simulink model "QCwithActDyn"  (R2019b)
settings: Solver=FixedStepAuto  StartTime=0.0  StopTime=15  FixedStep=0.001  RelTol=1e-3
model workspace (MAT data in the model file):
  time_step = 0.01
libraries: simulink x1
settings Model: Creator=Abdulaziz Y. Alkayas  LastModifiedBy=aaa_b
settings SolverCC: SolverResetMethod=Robust
settings DebuggingCC: ArithmeticOperatorsInVariantConditions=warning
settings HardwareCC: TargetBitPerPointer=64  TargetBitPerSizeT=64  TargetBitPerPtrDiffT=64  TargetLongLongMode=on  TargetIntDivRoundTo=Zero  TargetEndianess=LittleEndian  TargetWordSize=64  TargetHWDeviceType=MATLAB Host  ProdEqTarget=off
settings SFSimCC: CustomCodeUndefinedFunction=UseInterfaceOnly
settings RTWCC: Description=Generic Real-Time Target

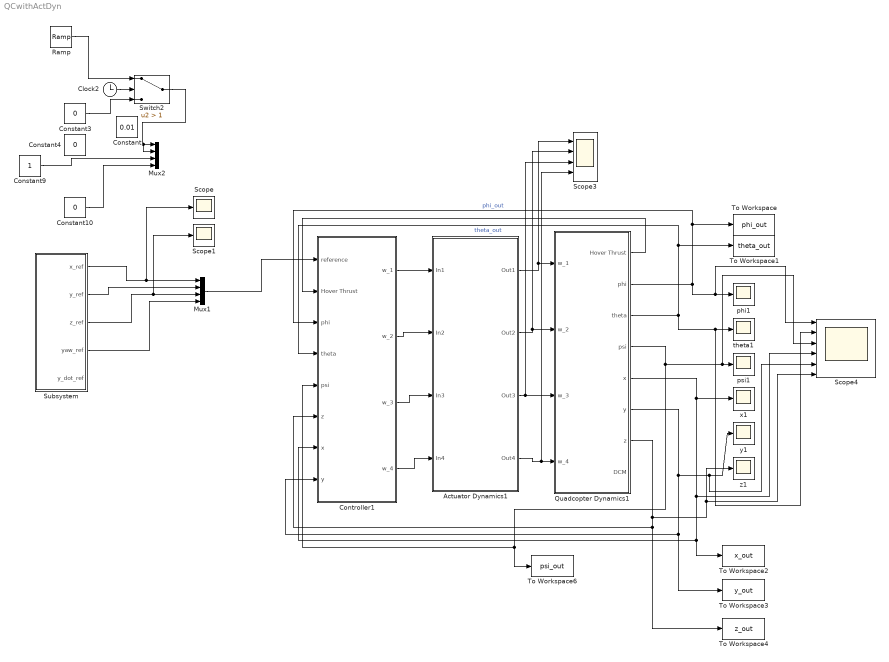
== system QCwithActDyn ==
  Actuator Dynamics1 : Subsystem
  Clock2 : Clock
  Constant : Constant  Value=0.01
  Constant10 : Constant  Value=0
  Constant3 : Constant  Value=0
  Constant4 : Constant  Value=0
  Constant9 : Constant
  Controller1 : Subsystem
  Mux1 : Mux
  Mux2 : Mux
  Quadcopter Dynamics1 : Subsystem
  Ramp : simulink/Sources/Ramp  slope=1  start=2  InitialOutput=0
  Scope : Scope
  Scope1 : Scope
  Scope3 : Scope  NumInputPorts=4
  Scope4 : Scope  NumInputPorts=6
  Subsystem : Subsystem
  Switch2 : Switch  Criteria=u2 > Threshold  Threshold=1
  To Workspace : ToWorkspace  VariableName=phi_out  SaveFormat=Timeseries  SampleTime=-1
  To Workspace1 : ToWorkspace  VariableName=theta_out  SaveFormat=Timeseries  SampleTime=-1
  To Workspace2 : ToWorkspace  VariableName=x_out  SaveFormat=Timeseries  SampleTime=-1
  To Workspace3 : ToWorkspace  VariableName=y_out  SaveFormat=Timeseries  SampleTime=-1
  To Workspace4 : ToWorkspace  VariableName=z_out  SaveFormat=Timeseries  SampleTime=-1
  To Workspace6 : ToWorkspace  VariableName=psi_out  SaveFormat=Timeseries  SampleTime=-1
  phi1 : Scope
  psi1 : Scope
  theta1 : Scope
  x1 : Scope
  y1 : Scope
  z1 : Scope
  wires:
  Controller1/4(w_4) -> Actuator Dynamics1/4(In4)
  Controller1/3(w_3) -> Actuator Dynamics1/3(In3)
  Controller1/2(w_2) -> Actuator Dynamics1/2(In2)
  Controller1/1(w_1) -> Actuator Dynamics1/1(In1)
  Quadcopter Dynamics1/3(theta) -> theta1/1, Scope4/2, To Workspace1/1, Controller1/4(theta)  "theta_out"
  Quadcopter Dynamics1/2(phi) -> Controller1/3(phi), To Workspace/1, phi1/1, Scope4/1  "phi_out"
  Quadcopter Dynamics1/4(psi) -> To Workspace6/1, Controller1/5(psi), psi1/1, Scope4/3
  Quadcopter Dynamics1/7(z) -> To Workspace4/1, Controller1/6(z), z1/1, Scope4/6
  Quadcopter Dynamics1/1(Hover Thrust) -> Controller1/2(Hover Thrust)
  Quadcopter Dynamics1/5(x) -> Scope4/4, To Workspace2/1, Controller1/7(x), x1/1
  Quadcopter Dynamics1/6(y) -> To Workspace3/1, Controller1/8(y), y1/1, Scope4/5
  Ramp/1 -> Switch2/1
  Constant9/1 -> Mux2/3
  Constant10/1 -> Mux2/4
  Clock2/1 -> Switch2/2
  Constant3/1 -> Switch2/3
  Subsystem/4("yaw_ref ") -> Mux1/4
  Subsystem/1("x_ref ") -> Mux1/1, Scope/1
  Switch2/1 -> Mux2/2, Mux2/1
  Mux1/1 -> Controller1/1(reference)
  Subsystem/3("z_ref ") -> Scope1/1, Mux1/3
  Actuator Dynamics1/1(Out1) -> Scope3/1, Quadcopter Dynamics1/1(w_1)
  Actuator Dynamics1/2(Out2) -> Quadcopter Dynamics1/2(w_2), Scope3/2
  Actuator Dynamics1/3(Out3) -> Quadcopter Dynamics1/3(w_3), Scope3/3
  Actuator Dynamics1/4(Out4) -> Quadcopter Dynamics1/4(w_4), Scope3/4
  Subsystem/2("y_ref ") -> Mux1/2

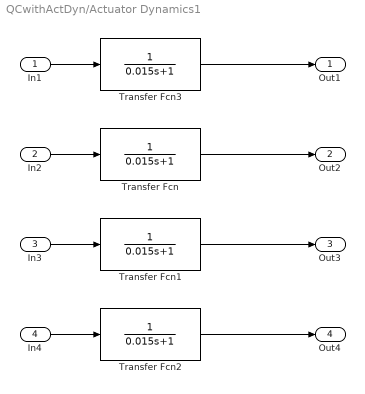
== system QCwithActDyn/Actuator Dynamics1 ==
  In1 : Inport
  In2 : Inport  Port=2
  In3 : Inport  Port=3
  In4 : Inport  Port=4
  Transfer Fcn{,1..3} (4 alike) : TransferFcn  Denominator=[0.015 1]
  Out1 : Outport
  Out2 : Outport  Port=2
  Out3 : Outport  Port=3
  Out4 : Outport  Port=4
  wires:
  In4/1 -> Transfer Fcn2/1
  Transfer Fcn2/1 -> Out4/1
  Transfer Fcn1/1 -> Out3/1
  In2/1 -> Transfer Fcn/1
  Transfer Fcn/1 -> Out2/1
  Transfer Fcn3/1 -> Out1/1
  In3/1 -> Transfer Fcn1/1
  In1/1 -> Transfer Fcn3/1

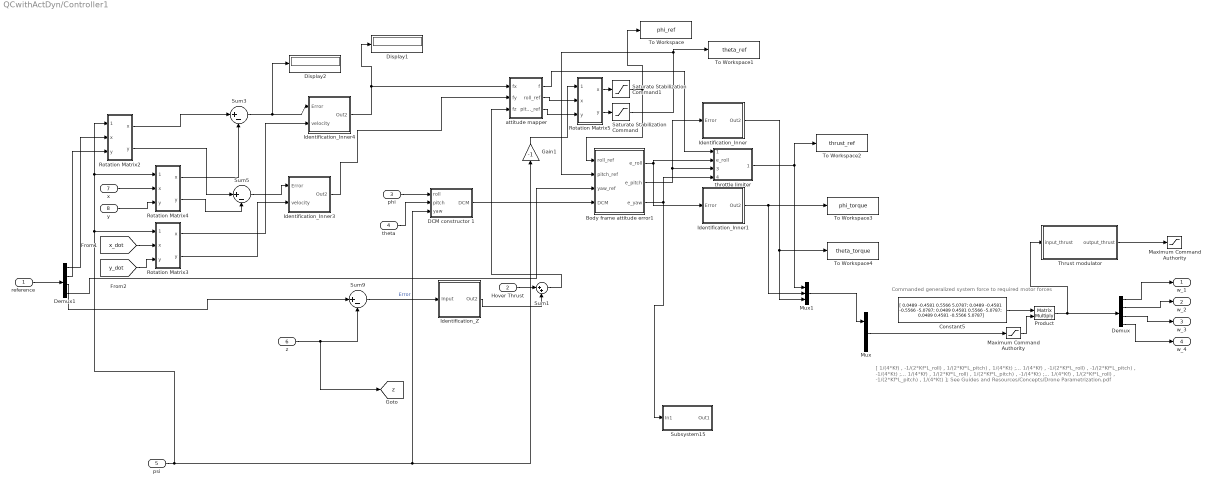
== system QCwithActDyn/Controller1 ==
  note: [ 1/(4*Kf) , -1/(2*Kf*L_roll) , 1/(2*Kf*L_pitch) , 1/(4*Kt) ;...
      | 1/(4*Kf) , -1/(2*Kf*L_roll) , -1/(2*Kf*L_pitch) , -1/(4*Kt) ;...
      | 1/(4*Kf) , 1/(2*Kf*L_roll) , 1/(2*Kf*L_pitch) , -1/(4*Kt) ;...
      | 1/(4*Kf) , 1/(2*Kf*L_roll) , -1/(2*Kf*L_pitch) , 1/(4*Kt) ];
      |
      | See Guides and Resources/Concepts/Drone Parametrization.pdf
  note: Commanded generalized system force to required motor forces
  reference : Inport
  Hover Thrust : Inport  Port=2
  phi : Inport  Port=3
  theta : Inport  Port=4
  psi : Inport  Port=5
  z : Inport  Port=6
  x : Inport  Port=7
  y : Inport  Port=8
  Body frame attitude error1 : MATLAB Function  TreatAsAtomicUnit=on
  Constant5 : Constant  Value=|
      | [ 0.0489   -0.4581    0.5566    5.0787;
      |   0.0489   -0.4581   -0.5566   -5.0787;
      |   0.0489    0.4581    0.5566   -5.0787;
      |   0.0489    0.4581   -0.5566    5.0787]
  DCM constructor 1 : MATLAB Function  TreatAsAtomicUnit=on
  Demux : Demux
  Demux1 : Demux
  Display1 : Display
  Display2 : Display
  Gain1 : Gain  Gain=-1
  Identification_Inner : Subsystem
  Identification_Inner1 : Subsystem
  Identification_Inner3 : Subsystem
  Identification_Inner4 : Subsystem
  Identification_Z : Subsystem
  Maximum Command Authority : Saturate  UpperLimit=[Inf Inf Inf Inf]  LowerLimit=[-inf -Inf -Inf -Inf]
  "Maximum Command Authority " : Saturate  UpperLimit=[1 1 1 1]  LowerLimit=[0 0 0 0]
  Mux : Mux  Inputs=[3, 1]
  Mux1 : Mux  Inputs=3
  Product : Product  Multiplication=Matrix(*)
  Rotation Matrix2 : Subsystem
  Rotation Matrix3 : Subsystem
  Rotation Matrix4 : Subsystem
  Rotation Matrix5 : Subsystem
  Saturate Stabilization Command : Saturate  UpperLimit=pi/2  LowerLimit=-pi/2
  Saturate Stabilization Command1 : Saturate  UpperLimit=pi/2  LowerLimit=-pi/2
  Subsystem15 : Subsystem
  Sum1 : Sum  Inputs=|++
  Sum3 : Sum  Inputs=|+-
  Sum5 : Sum  Inputs=|+-
  Sum9 : Sum  Inputs=|+-
  Thrust modulator : MATLAB Function  TreatAsAtomicUnit=on
  To Workspace : ToWorkspace  VariableName=phi_ref  SaveFormat=Timeseries  SampleTime=-1
  To Workspace1 : ToWorkspace  VariableName=theta_ref  SaveFormat=Timeseries  SampleTime=-1
  To Workspace2 : ToWorkspace  VariableName=thrust_ref  SaveFormat=Timeseries  SampleTime=-1
  To Workspace3 : ToWorkspace  VariableName=phi_torque  SaveFormat=Timeseries  SampleTime=-1
  To Workspace4 : ToWorkspace  VariableName=theta_torque  SaveFormat=Timeseries  SampleTime=-1
  "attitude mapper " : MATLAB Function  TreatAsAtomicUnit=on
  throttle limiter : MATLAB Function  TreatAsAtomicUnit=on
  w_1 : Outport
  w_2 : Outport  Port=2
  w_3 : Outport  Port=3
  w_4 : Outport  Port=4
  tag scope: z=global
  wires:
  z/1 -> Sum9/2, [z]
  Maximum Command Authority/1 -> Product/2
  Mux/1 -> Maximum Command Authority/1
  Constant5/1 -> Product/1
  Demux/2 -> w_2/1
  Demux/3 -> w_3/1
  Demux/4 -> w_4/1
  Sum3/1 -> Display2/1, Identification_Inner4/1(Error)
  Sum5/1 -> Identification_Inner3/1(Error)
  Hover Thrust/1 -> Sum1/1
  Demux/1 -> w_1/1
  Sum9/1 -> Identification_Z/1(Input)  "Error"
  Identification_Z/1(Out2) -> Sum1/2
  reference/1 -> Demux1/1
  Demux1/3 -> Sum9/1
  Identification_Inner4/1(Out2) -> Display1/1, "attitude mapper "/1(fx)
  Identification_Inner3/1(Out2) -> "attitude mapper "/2(fy)
  Sum1/1 -> "attitude mapper "/3(fz)
  Demux1/4 -> Body frame attitude error1/3(yaw_ref)
  Body frame attitude error1/3(e_yaw) -> throttle limiter/4(e_yaw), Subsystem15/1(In1)
  Body frame attitude error1/2(e_pitch) -> Identification_Inner/1(Error), throttle limiter/3(e_pitch)
  Body frame attitude error1/1(e_roll) -> Identification_Inner1/1(Error), throttle limiter/2(e_roll)
  Demux1/1 -> Rotation Matrix2/2("x ")
  Demux1/2 -> Rotation Matrix2/3(y)
  Rotation Matrix2/1(x) -> Sum3/1
  Rotation Matrix2/2("y ") -> Sum5/1
  [x_dot] -> Rotation Matrix3/2("x ")
  [y_dot] -> Rotation Matrix3/3(y)
  Rotation Matrix3/1(x) -> Identification_Inner4/2("velocity ")
  Rotation Matrix3/2("y ") -> Identification_Inner3/2("velocity ")
  x/1 -> Rotation Matrix4/2("x ")
  y/1 -> Rotation Matrix4/3(y)
  Rotation Matrix4/1(x) -> Sum3/2
  Rotation Matrix4/2("y ") -> Sum5/2
  DCM constructor 1/1(DCM) -> Body frame attitude error1/4(DCM)
  "attitude mapper "/2(roll_ref) -> Rotation Matrix5/2("x ")
  "attitude mapper "/3(pitch_ref) -> Rotation Matrix5/3(y)
  Rotation Matrix5/1(x) -> Saturate Stabilization Command1/1
  Identification_Inner1/1(Out2) -> Mux1/2, To Workspace3/1
  Identification_Inner/1(Out2) -> Mux1/3, To Workspace4/1
  Mux1/1 -> Mux/1
  psi/1 -> Rotation Matrix4/1("yaw "), Rotation Matrix2/1("yaw "), Rotation Matrix3/1("yaw "), Gain1/1, DCM constructor 1/3(yaw)
  Gain1/1 -> Rotation Matrix5/1("yaw ")
  Rotation Matrix5/2("y ") -> Saturate Stabilization Command/1
  Saturate Stabilization Command/1 -> To Workspace1/1, Body frame attitude error1/2(pitch_ref)
  Saturate Stabilization Command1/1 -> To Workspace/1, Body frame attitude error1/1(roll_ref)
  phi/1 -> DCM constructor 1/1(roll)
  theta/1 -> DCM constructor 1/2(pitch)
  "attitude mapper "/1(f) -> throttle limiter/1(throttle_in)
  throttle limiter/1(throttle_out) -> Mux1/1, To Workspace2/1
  Product/1 -> Thrust modulator/1(input_thrust), Demux/1
  Thrust modulator/1(output_thrust) -> "Maximum Command Authority "/1

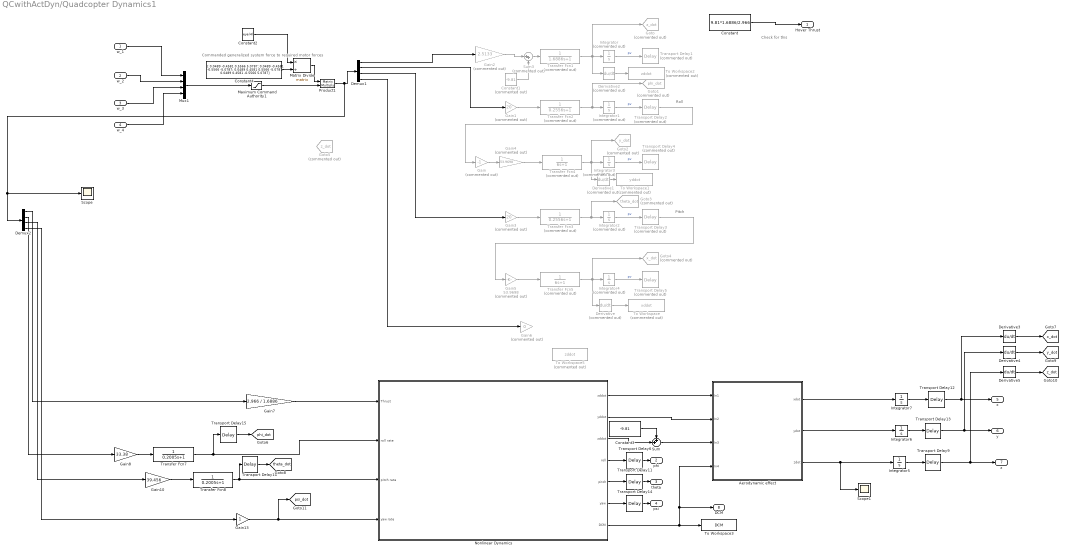
== system QCwithActDyn/Quadcopter Dynamics1 ==
  note: Check for this
  note: Pitch
  note: Roll
  note: Commanded generalized system force to required motor forces
  w_1 : Inport
  w_2 : Inport  Port=2
  w_3 : Inport  Port=3
  w_4 : Inport  Port=4
  "Aerodynamic effect " : Subsystem
  Constant : Constant  Value=9.81*1.6886/2.966
  Constant1 : Constant  Commented=on  Value=-9.81
  Constant2 : Constant  Value=eye(4)
  Constant3 : Constant  Value=-9.81
  Constant4 : Constant  Value=|
      | [ 0.0489   -0.4581    0.5566    5.0787;
      |   0.0489   -0.4581   -0.5566   -5.0787;
      |   0.0489    0.4581    0.5566   -5.0787;
      |   0.0489    0.4581   -0.5566    5.0787]
  Demux1 : Demux
  Demux2 : Demux
  Derivative : Derivative  Commented=on
  Derivative1 : Derivative  Commented=on
  Derivative2 : Derivative  Commented=on
  Derivative3 : Derivative
  Derivative4 : Derivative
  Derivative5 : Derivative
  Gain : Gain  Commented=on  Gain=-1
  Gain1 : Gain  Commented=on  Gain=20
  Gain10 : Gain  Gain=39.456
  Gain13 : Gain
  Gain2 : Gain  Commented=on  Gain=2.5133
  Gain3 : Gain  Commented=on  Gain=20
  Gain4 : Gain  Commented=on  Gain=53.9698
  Gain5 : Gain  Commented=on  Gain=53.9698
  Gain6 : Gain  Commented=on  Gain=0
  Gain7 : Gain  Gain=2.966 / 1.6886
  Gain8 : Gain  Gain=33.38
  Goto : Goto  Commented=on  GotoTag=z_dot  TagVisibility=global
  Goto1 : Goto  Commented=on  GotoTag=phi_dot  TagVisibility=global
  Goto2 : Goto  Commented=on  GotoTag=y_dot  TagVisibility=global
  Goto3 : Goto  Commented=on  GotoTag=theta_dot  TagVisibility=global
  Goto4 : Goto  Commented=on  GotoTag=x_dot  TagVisibility=global
  Goto5 : Goto  Commented=on  GotoTag=z_dot  TagVisibility=global
  Integrator{,1..4} (5 alike) : Integrator  Commented=on
  Integrator5 : Integrator
  Integrator6 : Integrator
  Integrator7 : Integrator  InitialCondition=-3
  Matrix Divide : Product  Inputs=*/  Multiplication=Matrix(*)
  Maximum Command Authority1 : Saturate  UpperLimit=[Inf Inf Inf Inf]  LowerLimit=[-Inf -Inf -Inf -Inf]
  Mux1 : Mux
  Nonlinear Dynamics : Subsystem
  Product1 : Product  Multiplication=Matrix(*)
  Scope : Scope
  Scope1 : Scope
  Sum : Sum  Inputs=++|
  Sum3 : Sum  Commented=on  Inputs=|++
  To Workspace : ToWorkspace  Commented=on  VariableName=xddot  SaveFormat=Timeseries  SampleTime=-1
  To Workspace1 : ToWorkspace  Commented=on  VariableName=yddot  SaveFormat=Timeseries  SampleTime=-1
  To Workspace2 : ToWorkspace  Commented=on  VariableName=zddot  SaveFormat=Timeseries  SampleTime=-1
  To Workspace3 : ToWorkspace  VariableName=DCM  SaveFormat=Timeseries  SampleTime=-1
  To Workspace5 : ToWorkspace  Commented=on  VariableName=zddot  SaveFormat=Timeseries  SampleTime=-1
  Transfer Fcn1 : TransferFcn  Commented=on  Denominator=[1.6886 1]
  Transfer Fcn2 : TransferFcn  Commented=on  Denominator=[0.2556 1]
  Transfer Fcn3 : TransferFcn  Commented=on  Denominator=[0.2556 1]
  Transfer Fcn4 : TransferFcn  Commented=on  Denominator=[6 1]
  Transfer Fcn5 : TransferFcn  Commented=on  Denominator=[6 1]
  Transfer Fcn7 : TransferFcn  Denominator=[0.2005 1]
  Transfer Fcn8 : TransferFcn  Denominator=[0.2005 1]
  Transport Delay1 : TransportDelay  Commented=on  DelayTime=0.0237
  Transport Delay{6,11,15..16} (4 alike) : TransportDelay  DelayTime=0.025
  Transport Delay12 : TransportDelay  DelayTime=0.0223  InitialOutput=-3
  Transport Delay13 : TransportDelay  DelayTime=0.0223
  Transport Delay14 : TransportDelay  DelayTime=0.01
  Transport Delay2 : TransportDelay  Commented=on  DelayTime=0.0180
  Transport Delay3 : TransportDelay  Commented=on  DelayTime=0.0180
  Transport Delay4 : TransportDelay  Commented=on  DelayTime=0.0223
  Transport Delay5 : TransportDelay  Commented=on  DelayTime=0.0223
  Transport Delay9 : TransportDelay  DelayTime=0.027
  Hover Thrust : Outport
  phi : Outport  Port=2
  theta : Outport  Port=3
  psi : Outport  Port=4
  x : Outport  Port=5
  y : Outport  Port=6
  z : Outport  Port=7
  DCM : Outport  Port=8
  tag scope: phi_dot=global, psi_dot=global, theta_dot=global, x_dot=global, y_dot=global, z_dot=global
  wires:
  Transfer Fcn1/1 -> Derivative2/1, Goto/1, Integrator/1
  Integrator/1 -> Transport Delay1/1  "pv"
  Integrator1/1 -> Transport Delay2/1  "pv"
  Transfer Fcn2/1 -> Goto1/1, Integrator1/1
  Gain1/1 -> Transfer Fcn2/1
  Transport Delay2/1 -> Gain/1
  Gain3/1 -> Transfer Fcn3/1
  Transfer Fcn3/1 -> Goto3/1, Integrator2/1
  Integrator2/1 -> Transport Delay3/1  "pv"
  Transport Delay3/1 -> Gain5/1
  Demux1/2 -> Gain1/1
  Demux1/3 -> Gain3/1
  Integrator3/1 -> Transport Delay4/1  "pv"
  Gain5/1 -> Transfer Fcn5/1
  Transfer Fcn5/1 -> Derivative/1, Goto4/1, Integrator4/1
  Sum3/1 -> Transfer Fcn1/1
  Integrator4/1 -> Transport Delay5/1  "pv"
  Demux1/4 -> Gain6/1
  w_2/1 -> Mux1/2
  w_3/1 -> Mux1/3
  w_4/1 -> Mux1/4
  Maximum Command Authority1/1 -> Product1/2
  Constant2/1 -> Matrix Divide/1
  Mux1/1 -> Maximum Command Authority1/1
  Constant4/1 -> Matrix Divide/2
  w_1/1 -> Mux1/1
  Demux1/1 -> Gain2/1
  Constant1/1 -> Sum3/2
  Gain2/1 -> Sum3/1
  Gain/1 -> Gain4/1
  Transfer Fcn4/1 -> Derivative1/1, Goto2/1, Integrator3/1
  Gain4/1 -> Transfer Fcn4/1
  Derivative/1 -> To Workspace/1
  Derivative1/1 -> To Workspace1/1
  Derivative2/1 -> To Workspace2/1
  Nonlinear Dynamics/1(xddot) -> "Aerodynamic effect "/1(In1)
  Nonlinear Dynamics/2(yddot) -> "Aerodynamic effect "/2(In2)
  Nonlinear Dynamics/7(DCM) -> To Workspace3/1, "Aerodynamic effect "/4(In4), DCM/1
  Integrator7/1 -> Transport Delay12/1
  Demux2/4 -> Gain13/1
  Demux2/3 -> Gain10/1
  Demux2/2 -> Gain8/1
  Transfer Fcn8/1 -> Transport Delay16/1, Nonlinear Dynamics/3(pitch rate)
  Gain10/1 -> Transfer Fcn8/1
  Gain8/1 -> Transfer Fcn7/1
  Nonlinear Dynamics/4(roll) -> Transport Delay6/1
  Nonlinear Dynamics/5("pitch ") -> Transport Delay11/1
  "Aerodynamic effect "/1("xdot ") -> Integrator7/1
  "Aerodynamic effect "/2(ydot) -> Integrator6/1
  Nonlinear Dynamics/3(zddot) -> Sum/2
  Sum/1 -> "Aerodynamic effect "/3(In3)
  Transport Delay11/1 -> theta/1
  Transport Delay6/1 -> phi/1
  Integrator5/1 -> Transport Delay9/1
  Transport Delay12/1 -> Derivative3/1, x/1
  Integrator6/1 -> Transport Delay13/1
  Transfer Fcn7/1 -> Transport Delay15/1, Nonlinear Dynamics/2("roll rate ")
  "Aerodynamic effect "/3(zdot) -> Scope1/1, Integrator5/1
  Constant3/1 -> Sum/1
  Constant/1 -> Hover Thrust/1
  Demux2/1 -> Gain7/1
  Transport Delay14/1 -> psi/1
  Nonlinear Dynamics/6(yaw) -> Transport Delay14/1
  Transport Delay15/1 -> [phi_dot]
  Transport Delay16/1 -> [theta_dot]
  Gain13/1 -> [psi_dot], Nonlinear Dynamics/4("yaw rate ")
  Gain7/1 -> Nonlinear Dynamics/1(Thrust)
  Derivative5/1 -> [z_dot]
  Derivative4/1 -> [y_dot]
  Transport Delay9/1 -> Derivative5/1, z/1
  Derivative3/1 -> [x_dot]
  Transport Delay13/1 -> Derivative4/1, y/1
  Product1/1 -> Scope/1, Demux2/1, Demux1/1
  Matrix Divide/1 -> Product1/1

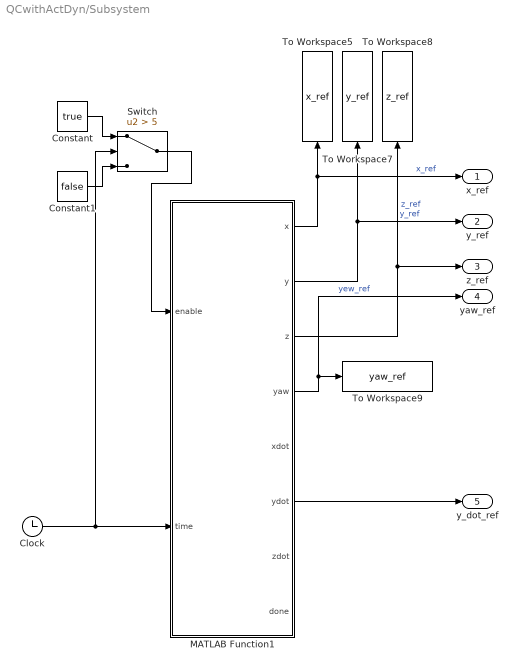
== system QCwithActDyn/Subsystem ==
  Clock : Clock
  Constant : Constant  Value=true
  Constant1 : Constant  Value=false
  MATLAB Function1 : MATLAB Function  TreatAsAtomicUnit=on
  Switch : Switch  Criteria=u2 > Threshold  Threshold=5
  To Workspace5 : ToWorkspace  VariableName=x_ref  SaveFormat=Timeseries  SampleTime=-1
  To Workspace7 : ToWorkspace  VariableName=y_ref  SaveFormat=Timeseries  SampleTime=-1
  To Workspace8 : ToWorkspace  VariableName=z_ref  SaveFormat=Timeseries  SampleTime=-1
  To Workspace9 : ToWorkspace  VariableName=yaw_ref  SaveFormat=Timeseries  SampleTime=-1
  "x_ref " : Outport
  "y_ref " : Outport  Port=2
  "z_ref " : Outport  Port=3
  "yaw_ref " : Outport  Port=4
  "y_dot_ref " : Outport  Port=5
  wires:
  Switch/1 -> MATLAB Function1/1(enable)
  Clock/1 -> Switch/2, MATLAB Function1/2(time)
  MATLAB Function1/3(z) -> To Workspace8/1, "z_ref "/1  "z_ref"
  MATLAB Function1/1(x) -> "x_ref "/1, To Workspace5/1  "x_ref"
  MATLAB Function1/2(y) -> "y_ref "/1, To Workspace7/1  "y_ref"
  MATLAB Function1/4(yaw) -> "yaw_ref "/1, To Workspace9/1  "yew_ref"
  Constant/1 -> Switch/1
  Constant1/1 -> Switch/3
  MATLAB Function1/6(ydot) -> "y_dot_ref "/1

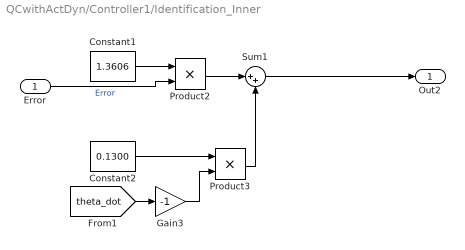
== system QCwithActDyn/Controller1/Identification_Inner ==
  Error : Inport
  Constant1 : Constant  Value=1.3606
  Constant2 : Constant  Value=0.1300
  Gain3 : Gain  Gain=-1
  Product2 : Product
  Product3 : Product
  Sum1 : Sum  Inputs=|++
  Out2 : Outport
  wires:
  Error/1 -> Product2/2  "Error"
  [theta_dot] -> Gain3/1
  Product2/1 -> Sum1/1
  Constant2/1 -> Product3/1
  Gain3/1 -> Product3/2
  Constant1/1 -> Product2/1
  Sum1/1 -> Out2/1
  Product3/1 -> Sum1/2

== system QCwithActDyn/Controller1/Identification_Inner1 ==
  Error : Inport
  Constant3 : Constant  Value=1.6910
  Constant4 : Constant  Value=0.1615
  Gain3 : Gain  Gain=-1
  Product2 : Product
  Product3 : Product
  Sum1 : Sum  Inputs=|++
  Out2 : Outport
  wires:
  Sum1/1 -> Out2/1
  Product3/1 -> Sum1/2
  Constant4/1 -> Product3/1
  Constant3/1 -> Product2/1
  [phi_dot] -> Gain3/1
  Gain3/1 -> Product3/2
  Product2/1 -> Sum1/1
  Error/1 -> Product2/2  "Error"

== system QCwithActDyn/Controller1/Identification_Inner3 ==
  Error : Inport
  "velocity " : Inport  Port=2
  Constant3 : Constant  Value=20.5475
  Constant4 : Constant  Value=6.8752
  Product2 : Product
  Product3 : Product
  Sum : Sum  Inputs=|-+
  Sum1 : Sum  Inputs=|++
  Out2 : Outport
  wires:
  Product2/1 -> Sum1/1
  Constant4/1 -> Product3/1
  Sum/1 -> Product3/2
  Constant3/1 -> Product2/1
  Sum1/1 -> Out2/1
  Product3/1 -> Sum1/2
  "velocity "/1 -> Sum/1  "Error"
  Error/1 -> Product2/2  "Error"

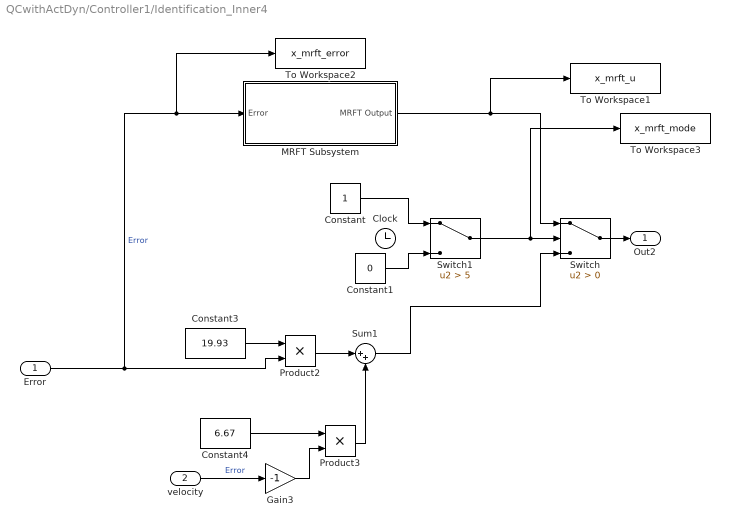
== system QCwithActDyn/Controller1/Identification_Inner4 ==
  Error : Inport
  "velocity " : Inport  Port=2
  Clock : Clock
  Constant : Constant
  Constant1 : Constant  Value=0
  Constant3 : Constant  Value=19.93
  Constant4 : Constant  Value=6.67
  Gain3 : Gain  Gain=-1
  MRFT Subsystem : Subsystem
  Product2 : Product
  Product3 : Product
  Sum1 : Sum  Inputs=|++
  Switch : Switch  Criteria=u2 > Threshold
  Switch1 : Switch  Criteria=u2 > Threshold  Threshold=5
  To Workspace1 : ToWorkspace  VariableName=x_mrft_u  SaveFormat=Timeseries  SampleTime=0.001
  To Workspace2 : ToWorkspace  VariableName=x_mrft_error  SaveFormat=Timeseries  SampleTime=0.001
  To Workspace3 : ToWorkspace  VariableName=x_mrft_mode  SaveFormat=Timeseries  SampleTime=0.001
  Out2 : Outport
  wires:
  Error/1 -> Product2/2, To Workspace2/1, MRFT Subsystem/1(Error)  "Error"
  Product2/1 -> Sum1/1
  Constant4/1 -> Product3/1
  Gain3/1 -> Product3/2
  Constant3/1 -> Product2/1
  Product3/1 -> Sum1/2
  Constant1/1 -> Switch1/3
  Constant/1 -> Switch1/1
  MRFT Subsystem/1(MRFT Output) -> To Workspace1/1, Switch/1
  Switch1/1 -> To Workspace3/1, Switch/2
  Sum1/1 -> Switch/3
  Switch/1 -> Out2/1
  "velocity "/1 -> Gain3/1  "Error"

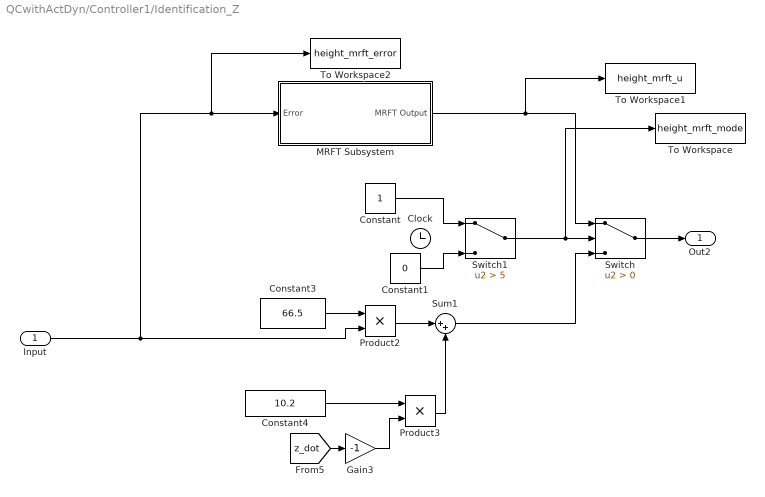
== system QCwithActDyn/Controller1/Identification_Z ==
  Input : Inport
  Clock : Clock
  Constant : Constant
  Constant1 : Constant  Value=0
  Constant3 : Constant  Value=66.5
  Constant4 : Constant  Value=10.2
  Gain3 : Gain  Gain=-1
  MRFT Subsystem : Subsystem
  Product2 : Product
  Product3 : Product
  Sum1 : Sum  Inputs=|++
  Switch : Switch  Criteria=u2 > Threshold
  Switch1 : Switch  Criteria=u2 > Threshold  Threshold=5
  To Workspace : ToWorkspace  VariableName=height_mrft_mode  SaveFormat=Timeseries  SampleTime=0.001
  To Workspace1 : ToWorkspace  VariableName=height_mrft_u  SaveFormat=Timeseries  SampleTime=0.001
  To Workspace2 : ToWorkspace  VariableName=height_mrft_error  SaveFormat=Timeseries  SampleTime=0.001
  Out2 : Outport
  wires:
  Constant4/1 -> Product3/1
  Gain3/1 -> Product3/2
  Product3/1 -> Sum1/2
  [z_dot] -> Gain3/1
  Product2/1 -> Sum1/1
  Constant3/1 -> Product2/1
  Input/1 -> To Workspace2/1, MRFT Subsystem/1(Error), Product2/2
  Switch/1 -> Out2/1
  Switch1/1 -> To Workspace/1, Switch/2
  Sum1/1 -> Switch/3
  MRFT Subsystem/1(MRFT Output) -> To Workspace1/1, Switch/1
  Constant1/1 -> Switch1/3
  Constant/1 -> Switch1/1

== system QCwithActDyn/Controller1/Rotation Matrix2 ==
  "yaw " : Inport
  "x " : Inport  Port=2
  y : Inport  Port=3
  reference correction : MATLAB Function  TreatAsAtomicUnit=on
  x : Outport
  "y " : Outport  Port=2
  wires:
  "yaw "/1 -> reference correction/1(yaw)
  "x "/1 -> reference correction/2(x)
  y/1 -> reference correction/3(y)
  reference correction/1(x_out) -> x/1
  reference correction/2(y_out) -> "y "/1

== system QCwithActDyn/Controller1/Rotation Matrix3 ==
  "yaw " : Inport
  "x " : Inport  Port=2
  y : Inport  Port=3
  reference correction : MATLAB Function  TreatAsAtomicUnit=on
  x : Outport
  "y " : Outport  Port=2
  wires:
  reference correction/2(y_out) -> "y "/1
  reference correction/1(x_out) -> x/1
  y/1 -> reference correction/3(y)
  "x "/1 -> reference correction/2(x)
  "yaw "/1 -> reference correction/1(yaw)

== system QCwithActDyn/Controller1/Rotation Matrix4 ==
  "yaw " : Inport
  "x " : Inport  Port=2
  y : Inport  Port=3
  reference correction : MATLAB Function  TreatAsAtomicUnit=on
  x : Outport
  "y " : Outport  Port=2
  wires:
  "yaw "/1 -> reference correction/1(yaw)
  "x "/1 -> reference correction/2(x)
  y/1 -> reference correction/3(y)
  reference correction/1(x_out) -> x/1
  reference correction/2(y_out) -> "y "/1

== system QCwithActDyn/Controller1/Rotation Matrix5 ==
  "yaw " : Inport
  "x " : Inport  Port=2
  y : Inport  Port=3
  reference correction : MATLAB Function  TreatAsAtomicUnit=on
  x : Outport
  "y " : Outport  Port=2
  wires:
  "yaw "/1 -> reference correction/1(yaw)
  "x "/1 -> reference correction/2(x)
  y/1 -> reference correction/3(y)
  reference correction/1(x_out) -> x/1
  reference correction/2(y_out) -> "y "/1

== system QCwithActDyn/Controller1/Subsystem15 ==
  In1 : Inport
  Gain2 : Gain  Gain=0.12
  Gain3 : Gain  Gain=0.6
  Sum6 : Sum  Inputs=|-+
  Out1 : Outport
  wires:
  Gain3/1 -> Sum6/2
  Gain2/1 -> Sum6/1
  Sum6/1 -> Out1/1
  In1/1 -> Gain3/1
  [psi_dot] -> Gain2/1

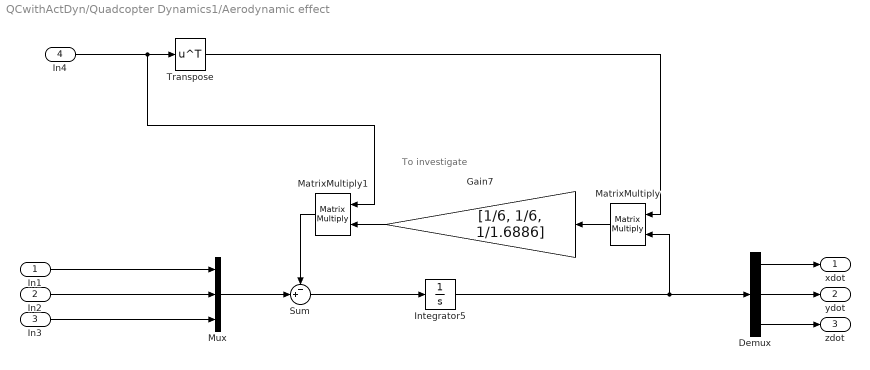
== system QCwithActDyn/Quadcopter Dynamics1/Aerodynamic effect  ==
  note: To investigate
  In1 : Inport
  In2 : Inport  Port=2
  In3 : Inport  Port=3
  In4 : Inport  Port=4
  Demux : Demux  Outputs=3
  Gain7 : Gain  Gain=[1/6, 1/6, 1/1.6886]
  Integrator5 : Integrator
  MatrixMultiply : Product  Multiplication=Matrix(*)
  MatrixMultiply1 : Product  Multiplication=Matrix(*)
  Mux : Mux  Inputs=3
  Sum : Sum  Inputs=-+|
  Transpose : Math  Operator=transpose  SignedPower=off  SaturateOnIntegerOverflow=on
  "xdot " : Outport
  ydot : Outport  Port=2
  zdot : Outport  Port=3
  wires:
  Mux/1 -> Sum/2
  In3/1 -> Mux/3
  MatrixMultiply/1 -> Gain7/1
  In2/1 -> Mux/2
  In1/1 -> Mux/1
  Demux/1 -> "xdot "/1
  Demux/2 -> ydot/1
  Demux/3 -> zdot/1
  Integrator5/1 -> MatrixMultiply/2, Demux/1
  Gain7/1 -> MatrixMultiply1/2
  Transpose/1 -> MatrixMultiply/1
  In4/1 -> MatrixMultiply1/1, Transpose/1
  Sum/1 -> Integrator5/1
  MatrixMultiply1/1 -> Sum/1

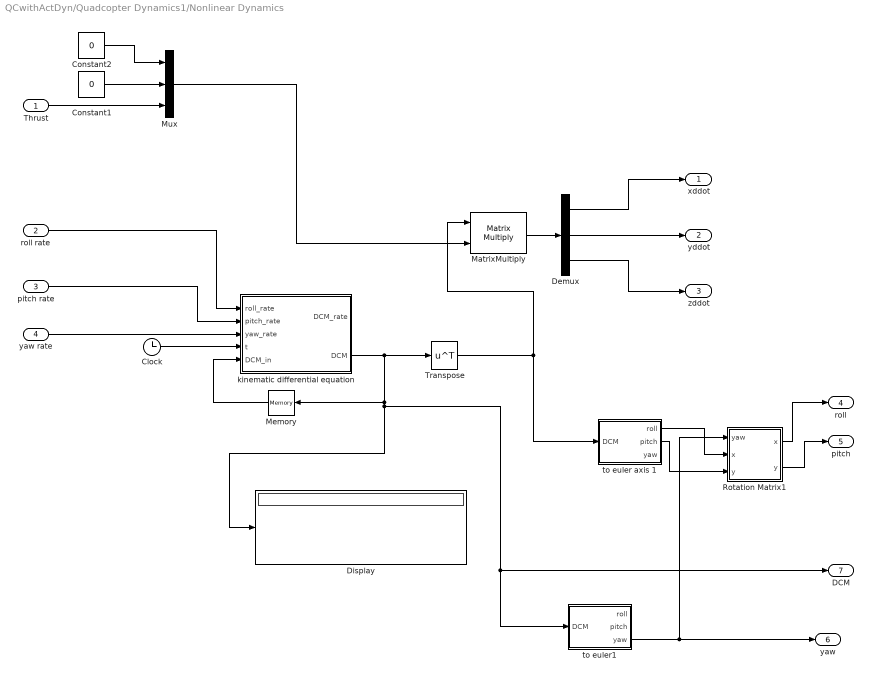
== system QCwithActDyn/Quadcopter Dynamics1/Nonlinear Dynamics ==
  Thrust : Inport
  "roll rate " : Inport  Port=2
  pitch rate : Inport  Port=3
  "yaw rate " : Inport  Port=4
  Clock : Clock
  Constant1 : Constant  Value=0
  Constant2 : Constant  Value=0
  Demux : Demux  Outputs=3
  Display : Display
  MatrixMultiply : Product  Multiplication=Matrix(*)
  Memory : Memory  InitialCondition=eye(3)
  Mux : Mux  Inputs=3
  Rotation Matrix1 : Subsystem
  Transpose : Math  Operator=transpose  SignedPower=off  SaturateOnIntegerOverflow=on
  kinematic differential equation : MATLAB Function  TreatAsAtomicUnit=on
  to euler axis 1 : MATLAB Function  TreatAsAtomicUnit=on
  to euler1 : MATLAB Function  TreatAsAtomicUnit=on
  xddot : Outport
  yddot : Outport  Port=2
  zddot : Outport  Port=3
  roll : Outport  Port=4
  "pitch " : Outport  Port=5
  yaw : Outport  Port=6
  DCM : Outport  Port=7
  wires:
  "yaw rate "/1 -> kinematic differential equation/3(yaw_rate)
  Thrust/1 -> Mux/3
  Constant2/1 -> Mux/1
  Constant1/1 -> Mux/2
  Mux/1 -> MatrixMultiply/2
  MatrixMultiply/1 -> Demux/1
  Demux/1 -> xddot/1
  Demux/2 -> yddot/1
  Demux/3 -> zddot/1
  "roll rate "/1 -> kinematic differential equation/1(roll_rate)
  pitch rate/1 -> kinematic differential equation/2(pitch_rate)
  Transpose/1 -> MatrixMultiply/1, to euler axis 1/1(DCM)
  to euler1/3(yaw) -> Rotation Matrix1/1("yaw "), yaw/1
  kinematic differential equation/2(DCM) -> Memory/1, to euler1/1(DCM), DCM/1, Display/1, Transpose/1
  Clock/1 -> kinematic differential equation/4(t)
  Memory/1 -> kinematic differential equation/5(DCM_in)
  to euler axis 1/1(roll) -> Rotation Matrix1/2("x ")
  to euler axis 1/2(pitch) -> Rotation Matrix1/3(y)
  Rotation Matrix1/2("y ") -> "pitch "/1
  Rotation Matrix1/1(x) -> roll/1

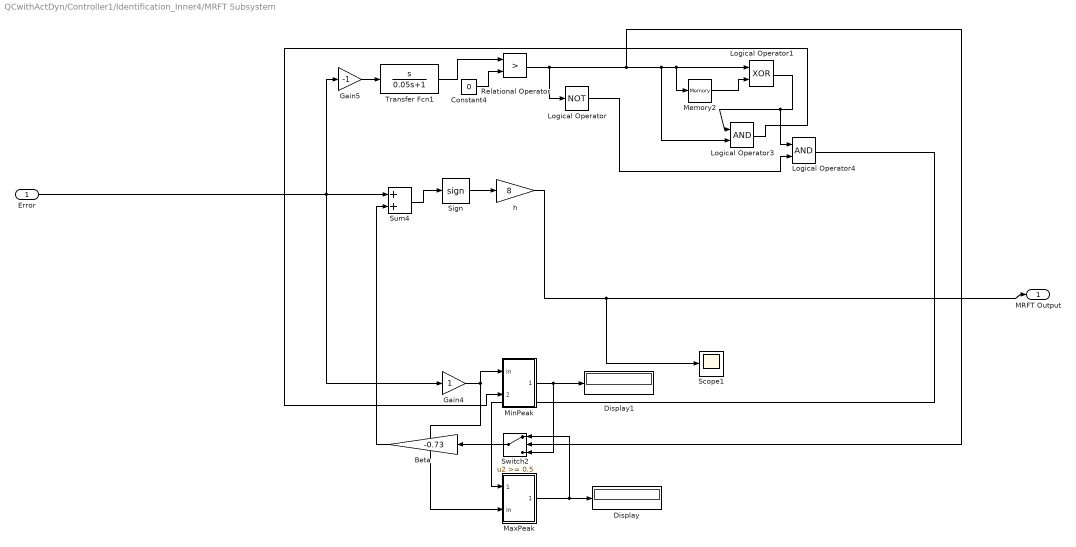
== system QCwithActDyn/Controller1/Identification_Inner4/MRFT Subsystem ==
  Error : Inport
  Beta : Gain  Gain=-0.73  SaturateOnIntegerOverflow=on  OutDataTypeStr=Inherit: Same as input  ParamDataTypeStr=Inherit: Same as input
  Constant4 : Constant  Value=0
  Display : Display
  Display1 : Display
  Gain4 : Gain  SaturateOnIntegerOverflow=on  OutDataTypeStr=Inherit: Same as input  ParamDataTypeStr=Inherit: Same as input
  Gain5 : Gain  Gain=-1  SaturateOnIntegerOverflow=on  OutDataTypeStr=Inherit: Same as input  ParamDataTypeStr=Inherit: Same as input
  Logical Operator : Logic  Operator=NOT  Inputs=1
  Logical Operator1 : Logic  Operator=XOR
  Logical Operator3 : Logic
  Logical Operator4 : Logic
  MaxPeak : Subsystem
  Memory2 : Memory
  MinPeak : Subsystem
  Relational Operator : RelationalOperator  Operator=>  RndMeth=Nearest  InputSameDT=on
  Scope1 : Scope
  Sign : Signum
  Sum4 : Sum  SaturateOnIntegerOverflow=on  InputSameDT=on  OutDataTypeStr=Inherit: Same as first input
  Switch2 : Switch  Threshold=0.5  SaturateOnIntegerOverflow=on  InputSameDT=on
  Transfer Fcn1 : TransferFcn  Numerator=[1 0]  Denominator=[0.05 1]
  h : Gain  Gain=8  SaturateOnIntegerOverflow=on  OutDataTypeStr=Inherit: Same as input  ParamDataTypeStr=Inherit: Same as input
  MRFT Output : Outport  VectorParamsAs1DForOutWhenUnconnected=off
  wires:
  MaxPeak/1(Out) -> Display/1, Switch2/1
  Beta/1 -> Sum4/2
  Error/1 -> Gain5/1, Sum4/1, Gain4/1
  Gain5/1 -> Transfer Fcn1/1
  Memory2/1 -> Logical Operator1/2
  Logical Operator3/1 -> MinPeak/2(Cntrl)
  Relational Operator/1 -> Logical Operator/1, Logical Operator1/1, Memory2/1, Logical Operator3/2, Switch2/2
  Sign/1 -> h/1
  Transfer Fcn1/1 -> Relational Operator/1
  Constant4/1 -> Relational Operator/2
  Gain4/1 -> MinPeak/1(In), MaxPeak/2(In)
  Switch2/1 -> Beta/1
  Sum4/1 -> Sign/1
  Logical Operator/1 -> Logical Operator4/2
  Logical Operator1/1 -> Logical Operator4/1, Logical Operator3/1
  Logical Operator4/1 -> MaxPeak/1(Cntrl)
  h/1 -> MRFT Output/1, Scope1/1
  MinPeak/1(Out) -> Display1/1, Switch2/3

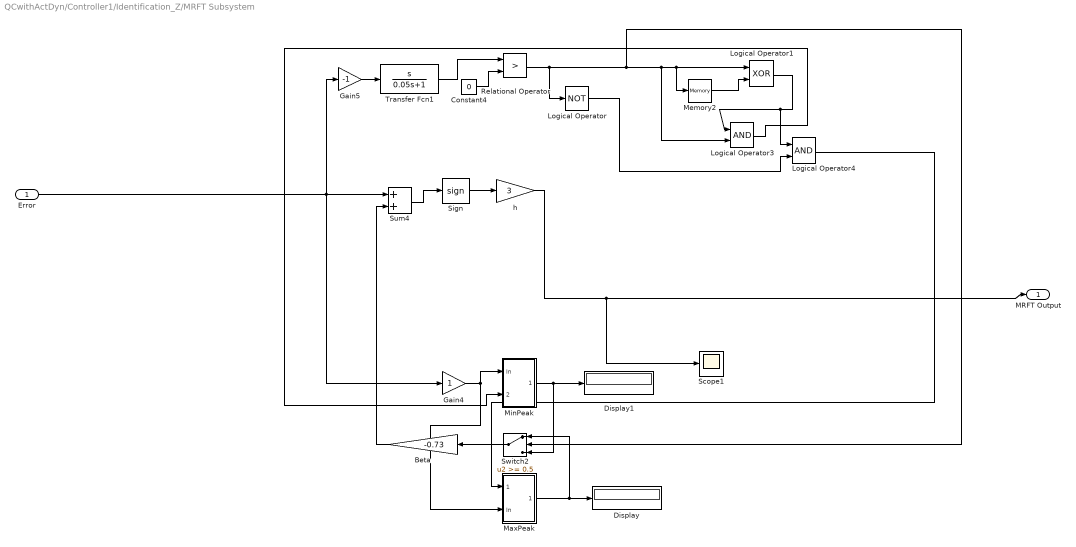
== system QCwithActDyn/Controller1/Identification_Z/MRFT Subsystem ==
  Error : Inport
  Beta : Gain  Gain=-0.73  SaturateOnIntegerOverflow=on  OutDataTypeStr=Inherit: Same as input  ParamDataTypeStr=Inherit: Same as input
  Constant4 : Constant  Value=0
  Display : Display
  Display1 : Display
  Gain4 : Gain  SaturateOnIntegerOverflow=on  OutDataTypeStr=Inherit: Same as input  ParamDataTypeStr=Inherit: Same as input
  Gain5 : Gain  Gain=-1  SaturateOnIntegerOverflow=on  OutDataTypeStr=Inherit: Same as input  ParamDataTypeStr=Inherit: Same as input
  Logical Operator : Logic  Operator=NOT  Inputs=1
  Logical Operator1 : Logic  Operator=XOR
  Logical Operator3 : Logic
  Logical Operator4 : Logic
  MaxPeak : Subsystem
  Memory2 : Memory
  MinPeak : Subsystem
  Relational Operator : RelationalOperator  Operator=>  RndMeth=Nearest  InputSameDT=on
  Scope1 : Scope
  Sign : Signum
  Sum4 : Sum  SaturateOnIntegerOverflow=on  InputSameDT=on  OutDataTypeStr=Inherit: Same as first input
  Switch2 : Switch  Threshold=0.5  SaturateOnIntegerOverflow=on  InputSameDT=on
  Transfer Fcn1 : TransferFcn  Numerator=[1 0]  Denominator=[0.05 1]
  h : Gain  Gain=3  SaturateOnIntegerOverflow=on  OutDataTypeStr=Inherit: Same as input  ParamDataTypeStr=Inherit: Same as input
  MRFT Output : Outport  VectorParamsAs1DForOutWhenUnconnected=off
  wires:
  MaxPeak/1(Out) -> Display/1, Switch2/1
  Beta/1 -> Sum4/2
  Error/1 -> Gain5/1, Sum4/1, Gain4/1
  Gain5/1 -> Transfer Fcn1/1
  Memory2/1 -> Logical Operator1/2
  Logical Operator3/1 -> MinPeak/2(Cntrl)
  Relational Operator/1 -> Logical Operator/1, Logical Operator1/1, Memory2/1, Logical Operator3/2, Switch2/2
  Sign/1 -> h/1
  Transfer Fcn1/1 -> Relational Operator/1
  Constant4/1 -> Relational Operator/2
  Gain4/1 -> MinPeak/1(In), MaxPeak/2(In)
  Switch2/1 -> Beta/1
  Sum4/1 -> Sign/1
  Logical Operator/1 -> Logical Operator4/2
  Logical Operator1/1 -> Logical Operator4/1, Logical Operator3/1
  Logical Operator4/1 -> MaxPeak/1(Cntrl)
  h/1 -> MRFT Output/1, Scope1/1
  MinPeak/1(Out) -> Display1/1, Switch2/3

== system QCwithActDyn/Quadcopter Dynamics1/Nonlinear Dynamics/Rotation Matrix1 ==
  "yaw " : Inport
  "x " : Inport  Port=2
  y : Inport  Port=3
  reference correction : MATLAB Function  TreatAsAtomicUnit=on
  x : Outport
  "y " : Outport  Port=2
  wires:
  reference correction/2(y_out) -> "y "/1
  reference correction/1(x_out) -> x/1
  y/1 -> reference correction/3(y)
  "x "/1 -> reference correction/2(x)
  "yaw "/1 -> reference correction/1(yaw)

== system QCwithActDyn/Controller1/Identification_Inner4/MRFT Subsystem/MaxPeak ==
  Cntrl : Inport
  In : Inport  Port=2
  Constant2 : Constant  Value=0
  Memory : Memory
  MinMax : MinMax  Function=max  Inputs=2  SaturateOnIntegerOverflow=on  InputSameDT=on
  Switch : Switch  Threshold=0.5  SaturateOnIntegerOverflow=on  InputSameDT=on
  Out : Outport  VectorParamsAs1DForOutWhenUnconnected=off
  wires:
  MinMax/1 -> Memory/1, Out/1
  Switch/1 -> MinMax/1
  Constant2/1 -> Switch/1
  Memory/1 -> Switch/3
  In/1 -> MinMax/2
  Cntrl/1 -> Switch/2

== system QCwithActDyn/Controller1/Identification_Inner4/MRFT Subsystem/MinPeak ==
  In : Inport
  Cntrl : Inport  Port=2
  Constant3 : Constant  Value=0
  Memory1 : Memory
  MinMax1 : MinMax  Inputs=2  SaturateOnIntegerOverflow=on  InputSameDT=on
  Switch1 : Switch  Threshold=0.5  SaturateOnIntegerOverflow=on  InputSameDT=on
  Out : Outport  VectorParamsAs1DForOutWhenUnconnected=off
  wires:
  MinMax1/1 -> Memory1/1, Out/1
  Switch1/1 -> MinMax1/2
  Memory1/1 -> Switch1/3
  Constant3/1 -> Switch1/1
  In/1 -> MinMax1/1
  Cntrl/1 -> Switch1/2

== system QCwithActDyn/Controller1/Identification_Z/MRFT Subsystem/MaxPeak ==
  Cntrl : Inport
  In : Inport  Port=2
  Constant2 : Constant  Value=0
  Memory : Memory
  MinMax : MinMax  Function=max  Inputs=2  SaturateOnIntegerOverflow=on  InputSameDT=on
  Switch : Switch  Threshold=0.5  SaturateOnIntegerOverflow=on  InputSameDT=on
  Out : Outport  VectorParamsAs1DForOutWhenUnconnected=off
  wires:
  MinMax/1 -> Memory/1, Out/1
  Switch/1 -> MinMax/1
  Constant2/1 -> Switch/1
  Memory/1 -> Switch/3
  In/1 -> MinMax/2
  Cntrl/1 -> Switch/2

== system QCwithActDyn/Controller1/Identification_Z/MRFT Subsystem/MinPeak ==
  In : Inport
  Cntrl : Inport  Port=2
  Constant3 : Constant  Value=0
  Memory1 : Memory
  MinMax1 : MinMax  Inputs=2  SaturateOnIntegerOverflow=on  InputSameDT=on
  Switch1 : Switch  Threshold=0.5  SaturateOnIntegerOverflow=on  InputSameDT=on
  Out : Outport  VectorParamsAs1DForOutWhenUnconnected=off
  wires:
  MinMax1/1 -> Memory1/1, Out/1
  Switch1/1 -> MinMax1/2
  Memory1/1 -> Switch1/3
  Constant3/1 -> Switch1/1
  In/1 -> MinMax1/1
  Cntrl/1 -> Switch1/2

== matlab function QCwithActDyn/Subsystem/MATLAB Function1 ==
  settings: updateMethod=DISCRETE
  data: enable input; x output; time input; y output; z output; yaw output; xdot output; ydot output; zdot output; done output
function [x, y, z, yaw, xdot, ydot, zdot, done]= fcn(enable, time)

persistent start_time
persistent poly_x
persistent poly_y
persistent poly_z
persistent n_order
persistent ts
persistent trajectory_segment
persistent state 
%states:
%   1: First trajectory
%   2: Second trajectory
%   3: Third trajectory


if isempty(start_time) || isempty(trajectory_segment) || ~enable || isempty(state)
    start_time = time;
    trajectory_segment = 1;
    state = 1;
end

% if isempty(poly_x) || isempty(poly_y) || isempty(poly_z) || isempty(ts)
%     g = coder.load('8shape-15_time_minsnap.mat');
%     poly_t = g.y;
%     n_order = g.poly_order;
%     ts = g.T;
% end
% 
% T = 5.5;
% x = 0; y = 0; z = 1; yaw=0; done=false;
% xdot = 0; ydot = 0; zdot = 0; 
% if enable
%     t = time - start_time;
%     if t > T
%         x = 0; y = 0; z = 1; yaw = 0; done = true;
%         xdot = 0; ydot = 0; zdot = 0; 
%         return;
%     end
%     t_now = 0;
%     for i=0:n_order-1
%         t_now = t_now + poly_t(i+1) * t^i;
%     end
%     t_now = 2*pi*t_now/T - pi/2;
%     x = 1*cos(t_now)*sin(t_now);
%     y = 1*cos(t_now);
%     
% end



% if isempty(poly_x) || isempty(poly_y) || isempty(poly_z) || isempty(ts)
%     g = coder.load('90_deg_roll24.mat');
%     poly_x = g.polys_x;
%     poly_y = g.polys_y;
%     poly_z = g.polys_z;
%     n_order = g.n_order(1);
%     ts = g.ts;
% end
% 
% x = -3; y = 0; z = 0.75; yaw=0; done=false;
% xdot = 0; ydot = 0; zdot = 0; 
% if enable
%     t = time - start_time;
%     if t > ts(end)
%         t=ts(end)
%     elseif t > ts(trajectory_segment + 1)
%         trajectory_segment = trajectory_segment + 1;
%     end
% 
% %     poly_x_i = poly_x(:, trajectory_segment);
% %     poly_y_i = poly_y(:, trajectory_segment);
% %     poly_z_i = poly_z(:, trajectory_segment);
%     poly_x_i = poly_x{trajectory_segment};
%     poly_y_i = poly_y{trajectory_segment};
%     poly_z_i = poly_z{trajectory_segment};
% 
%     x = 0; y = 0; z = 0.15;
%     for i=0:n_order
%         x = x + poly_x_i(i+1) * t^i;
%         y = y + poly_y_i(i+1) * t^i;
%         z = z + poly_z_i(i+1) * t^i;
%         if i>0
%             xdot = xdot + i * poly_x_i(i+1) * t^(i-1);
%             ydot = ydot + i * poly_y_i(i+1) * t^(i-1);
%             zdot = zdot + i * poly_z_i(i+1) * t^(i-1);
%         end
%     end
% end


if isempty(poly_x) || isempty(poly_y) || isempty(poly_z) || isempty(n_order) || isempty(ts)
    g = coder.load('90_deg_roll24.mat');
    poly_x = g.polys_x;
    poly_y = g.polys_y;
    poly_z = g.polys_z;
    n_order = g.n_order(1);
    ts = g.ts;
end


x = -3; y = 0; z = 0.75; yaw=0; done=false;
xdot = 0; ydot = 0; zdot = 0; 
if enable
    t = time - start_time; 
    tt = t;
    if t > ts(end)
        tt = ts(end);
    elseif t > ts(trajectory_segment + 1)
        trajectory_segment = trajectory_segment + 1;
    end

%     poly_x_i = poly_x(:, trajectory_segment);
%     poly_y_i = poly_y(:, trajectory_segment);
%     poly_z_i = poly_z(:, trajectory_segment);
    poly_x_i = poly_x{trajectory_segment};
    poly_y_i = poly_y{trajectory_segment};
    poly_z_i = poly_z{trajectory_segment};

    offset = [0, 0, 0];
    if state == 1
        offset = [0, 0, 0.15];
    elseif state == 2
        offset = [0, 0, 0.15];
    elseif state == 3
        offset = [-0.25, 0.2, 0.25];
    end
    x = offset(1); y = offset(2); z = offset(3);
    for i=0:n_order
        x = x + poly_x_i(i+1) * tt^i;
        y = y + poly_y_i(i+1) * tt^i;
        z = z + poly_z_i(i+1) * tt^i;
        if i>0
            xdot = xdot + i * poly_x_i(i+1) * tt^(i-1);
            ydot = ydot + i * poly_y_i(i+1) * tt^(i-1);
            zdot = zdot + i * poly_z_i(i+1) * tt^(i-1);
        end
    end
    
    if t > ts(end)+0.5
        switch state
            case 1
                state = 2;
                start_time = time;
                g = coder.load('reset_traj_24_16.mat');
                poly_x = g.polys_x;
                poly_y = g.polys_y;
                poly_z = g.polys_z;
                n_order = g.n_order(1);
                ts = g.ts;
                trajectory_segment = 1;
            case 2
                if t > ts(end)+6
                    state = 3;
                    start_time = time;
                    g = coder.load('90_deg_roll16.mat');                
                    poly_x = g.polys_x;
                    poly_y = g.polys_y;
                    poly_z = g.polys_z;
                    n_order = g.n_order(1);
                    ts = g.ts;     
                    trajectory_segment = 1;       
                end
                
        end
    end
        
end

== matlab function QCwithActDyn/Quadcopter Dynamics1/Nonlinear Dynamics/kinematic differential equation ==
  settings: updateMethod=DISCRETE
  data: roll_rate input; DCM_rate output; pitch_rate input; yaw_rate input; t input; DCM_in input; DCM output
function [DCM_rate, DCM]  = fcn(roll_rate, pitch_rate, yaw_rate, t, DCM_in)

persistent last_t;

if isempty(last_t)
    last_t = 0;
end

omega_tilde = [0, -yaw_rate, pitch_rate;
               yaw_rate, 0, -roll_rate;
               -pitch_rate, roll_rate, 0];
DCM_rate = - omega_tilde * DCM_in;

DCM = DCM_in + DCM_rate * (t-last_t);

DCM = DCM / nthroot(det(DCM), 3);

last_t = t;

if abs(roll_rate)>0
   pose=1;
end

== matlab function QCwithActDyn/Quadcopter Dynamics1/Nonlinear Dynamics/Rotation Matrix1/reference correction ==
  data: yaw input; x_out output; x input; y input; y_out output
function [x_out,y_out] = fcn(yaw, x, y)

dcm = [cos(yaw) sin(yaw); -sin(yaw) cos(yaw)];

out = dcm * [x; y];
x_out = out(1);
y_out = out(2);

== matlab function QCwithActDyn/Controller1/attitude mapper  ==
  data: fx input; f output; fy input; fz input; roll_ref output; pitch_ref output
function [f, roll_ref, pitch_ref] = fcn(fx, fy, fz)

if fz>0
    f = sqrt(fx*fx + fy*fy + fz*fz);
else
    f = sqrt(fx*fx + fy*fy + 0);
end

unit_x_vector = [1, 0, 0];
unit_y_vector = [0, 1, 0];
unit_z_vector = [0, 0, 1];

if f == 0
    roll_ref = 0;
    pitch_ref = 0;    
else
    fz=abs(fz);
    force_vector = [fx, fy, fz];
    theta = acos(dot(unit_z_vector, force_vector) / norm(force_vector));
    
    if theta==0
        roll_ref = 0;
        pitch_ref = 0; 
    else        
        force_xy_projection = [fx; fy] / norm([fx; fy]);
        rotation_vector = [cos(pi/2) -sin(pi/2); sin(pi/2) cos(pi/2)] * force_xy_projection;
        roll_ref = theta * rotation_vector(1);
        pitch_ref = theta * rotation_vector(2);
    end
end

end

== matlab function QCwithActDyn/Controller1/Rotation Matrix2/reference correction ==
  data: yaw input; x_out output; x input; y input; y_out output
function [x_out,y_out] = fcn(yaw, x, y)

dcm = [cos(yaw) sin(yaw); -sin(yaw) cos(yaw)];

out = dcm * [x; y];
x_out = out(1);
y_out = out(2);

== matlab function QCwithActDyn/Quadcopter Dynamics1/Nonlinear Dynamics/to euler1 ==
  data: roll output; DCM input; pitch output; yaw output
function [roll, pitch, yaw] = fcn(DCM)

eul = rotm2eul(DCM);

yaw = eul(1);
pitch = eul(2);
roll = eul(3);

epsilon = 1e-2;
if abs(yaw)>epsilon
    g=1;
end
if(abs(pitch) >= (pi/2 - epsilon) && abs(yaw) > 0)
    %singularity
    roll = yaw + roll;
    while(abs(roll) >= pi - epsilon)
        roll = roll - sign(roll) * pi;
    end
    yaw = 0;
end

== matlab function QCwithActDyn/Quadcopter Dynamics1/Nonlinear Dynamics/to euler axis 1 ==
  data: roll output; DCM input; pitch output; yaw output
function [roll, pitch, yaw] = fcn(DCM)

g = trace((trace(DCM) - 1) / 2);
g = min(1, max(g, -1));
theta = acos(g);

if(theta ~= 0)
    roll = theta * ( DCM(3,2) - DCM(2,3) ) / (2 * sin(theta));
    pitch = theta * ( DCM(1,3) - DCM(3,1) ) / (2 * sin(theta));
    yaw = theta * ( DCM(2,1) - DCM(1,2) ) / (2 * sin(theta));
else
    roll = 0;
    pitch = 0;
    yaw = 0;
end

== matlab function QCwithActDyn/Controller1/Body frame attitude error1 ==
  data: roll_ref input; pitch_ref input; yaw_ref input; e_roll output; e_pitch output; e_yaw output; DCM input
function [e_roll, e_pitch, e_yaw] = fcn(roll_ref, pitch_ref, yaw_ref, DCM)

DCM_yaw_ref = [cos(yaw_ref), -sin(yaw_ref), 0;
                sin(yaw_ref), cos(yaw_ref), 0;
                0, 0, 1];

yaw_ref = 0;
theta_ref = norm([roll_ref, pitch_ref, yaw_ref]);

if(theta_ref ~= 0)
    euler_axis_ref = [roll_ref, pitch_ref, yaw_ref] / theta_ref;
else
    euler_axis_ref = [0, 0, 0];
end

%limit theta_ref
theta_ref = min(pi/2, max(theta_ref, -pi/2));

quaternion_ref = euler_axis_ref * sin(theta_ref / 2);
quaternion_ref = [cos(theta_ref / 2), quaternion_ref];

DCM_ref = DCM_yaw_ref * quat2rotm(quaternion_ref);

DCM_error = transpose(DCM) * DCM_ref;

g = trace((trace(DCM_error) - 1) / 2);
g = min(1, max(g, -1));
theta_error = acos(g);

if(theta_error ~= 0)
    e_roll = theta_error * ( DCM_error(3,2) - DCM_error(2,3) ) / (2 * sin(theta_error));
    e_pitch = theta_error * ( DCM_error(1,3) - DCM_error(3,1) ) / (2 * sin(theta_error));
    e_yaw = theta_error * ( DCM_error(2,1) - DCM_error(1,2) ) / (2 * sin(theta_error));
else
    e_roll = 0;
    e_pitch = 0;
    e_yaw = 0;
end


end

== matlab function QCwithActDyn/Controller1/Rotation Matrix3/reference correction ==
  data: yaw input; x_out output; x input; y input; y_out output
function [x_out,y_out] = fcn(yaw, x, y)

dcm = [cos(yaw) sin(yaw); -sin(yaw) cos(yaw)];

out = dcm * [x; y];
x_out = out(1);
y_out = out(2);

== matlab function QCwithActDyn/Controller1/Rotation Matrix4/reference correction ==
  data: yaw input; x_out output; x input; y input; y_out output
function [x_out,y_out] = fcn(yaw, x, y)

dcm = [cos(yaw) sin(yaw); -sin(yaw) cos(yaw)];

out = dcm * [x; y];
x_out = out(1);
y_out = out(2);

== matlab function QCwithActDyn/Controller1/DCM constructor 1 ==
  data: roll input; DCM output; pitch input; yaw input
function DCM = fcn(roll, pitch, yaw)

%DCM of yaw
yaw_DCM = [cos(yaw) -sin(yaw) 0;
            sin(yaw) cos(yaw) 0;
            0 0 1];
        
% pitch_DCM = [cos(pitch) 0 sin(pitch);
%             0, 1, 0;
%             -sin(pitch) 0 cos(pitch)];
%         
% roll_DCM = [1, 0, 0;
%             0 cos(yaw) -sin(roll);
%             0 sin(roll) cos(roll)];
%      
% DCM = yaw_DCM * pitch_DCM * roll_DCM;


% DCM of roll/pitch
theta_err = norm([roll, pitch, 0]);
euler_axis_err = [0, 0, 0];
if(theta_err ~= 0)
    euler_axis_err = [roll, pitch, 0] / theta_err;
end
%limit theta_ref
theta_err = min(pi/2, max(theta_err, -pi/2));
quaternion_err = euler_axis_err * sin(theta_err / 2);
quaternion_err = [cos(theta_err / 2), quaternion_err];
roll_pitch_DCM = quat2rotm(quaternion_err);


DCM = yaw_DCM * roll_pitch_DCM;

end

== matlab function QCwithActDyn/Controller1/Rotation Matrix5/reference correction ==
  data: yaw input; x_out output; x input; y input; y_out output
function [x_out,y_out] = fcn(yaw, x, y)

dcm = [cos(yaw) sin(yaw); -sin(yaw) cos(yaw)];

out = dcm * [x; y];
x_out = out(1);
y_out = out(2);

== matlab function QCwithActDyn/Controller1/Thrust modulator ==
  data: input_thrust input; output_thrust output
function output_thrust = fcn(input_thrust)

output_thrust = input_thrust;
if max(input_thrust) > 1
    output_thrust = input_thrust - max(input_thrust) + 1;
elseif min(input_thrust) < 0.05
    output_thrust = input_thrust - min(input_thrust) + 0.05;
end

== matlab function QCwithActDyn/Controller1/throttle limiter ==
  data: throttle_in input; e_roll input; e_pitch input; e_yaw input; throttle_out output
function throttle_out = fcn(throttle_in, e_roll, e_pitch, e_yaw)

throttle_out = throttle_in * cos(norm([e_roll, e_pitch, e_yaw]));

if (throttle_out < 0) 
    throttle_out = 0;
end
